simulink model "Ninebussys_Final"  (R2023b)
settings: Solver=FixedStepDiscrete  StartTime=0.0  StopTime=0.7  RelTol=1e-3
undefined symbols (not defined in the file or in its folder): D1, Delta
libraries: spsFourierLib x18, spsThreePhaseVIMeasurementLib x9, spsLoadFlowBusLib x9, spsPower3phInstantaneousLib x9, spsThreePhasePISectionLineLib x6, spsThreePhaseSeriesRLCLoadLib x4, spsThreePhaseTransformerTwoWindingsLib x3, spsSynchronousMachinepuStandardLib x3, spsThreePhaseParallelRLCLoadLib x3, spsExcitationSystemLib x3, spsGenericPowerSystemStabilizerLib x3, spsHydraulicTurbineandGovernorLib x3
settings Model: Creator=z0034ktr  LastModifiedBy=HP
settings SolverCC: AlgebraicLoopSolver=TrustRegion
settings DebuggingCC: UnconnectedInputMsg=warning  UnconnectedOutputMsg=warning  UnconnectedLineMsg=warning  ArithmeticOperatorsInVariantConditions=warning
settings ModelReferenceCC: EnableRefExpFcnMdlSchedulingChecks=on
settings SFSimCC: CustomCodeUndefinedFunction=UseInterfaceOnly

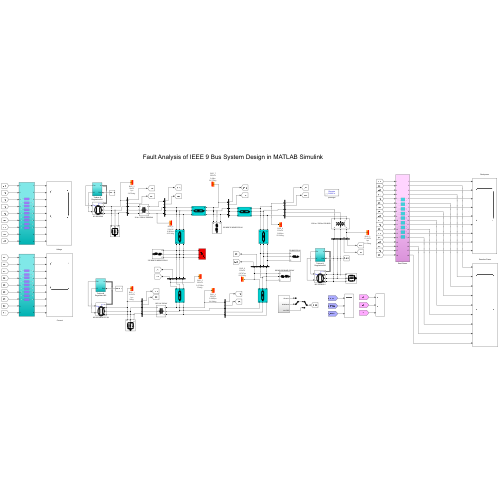
[thumbnail: Simulink's stored preview of the top-level diagram]
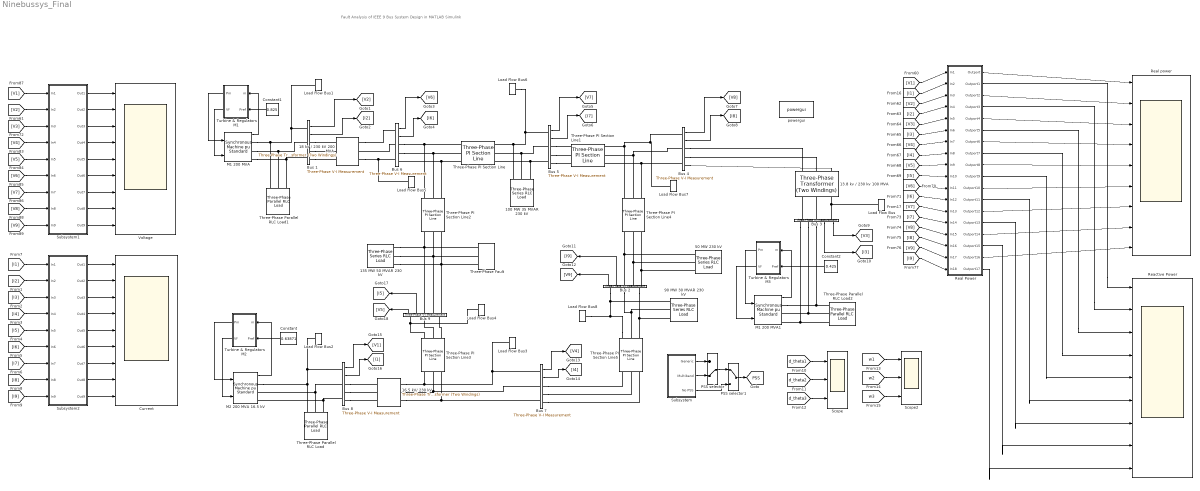
== system Ninebussys_Final ==
  note: Fault Analysis of IEEE 9 Bus System Design in MATLAB Simulink
  " Current" : Scope  NumInputPorts=9
  " Voltage" : Scope  NumInputPorts=9
  100 MW 35 MVAR 230 kV : spsThreePhaseSeriesRLCLoadLib/Three-Phase Series RLC Load  LConnTagsString=A|B|C  Configuration=Y (grounded)  NominalVoltage=(230000)*0.980041  Vabc=[1e3 1e3 1e3]  Vabcp=[1e3 1e3 1e3]  NominalFrequency=60  UnbalancedPower=off  ActivePower=100e6  InductivePower=35e6  CapacitivePower=0  Pabc=[10e3 9e3 11e3]  QLabc=[100 90 110]  QCabc=[100 90 110]  Pabcp=[10e3 9e3 11e3]  QLabcp=[100 90 110]  QCabcp=[100 90 110]  Measurements=None  LoadType=constant PQ
  13.8 kv / 230 kv 100 MVA : spsThreePhaseTransformerTwoWindingsLib/Three-Phase Transformer (Two Windings)  Winding1Connection=Delta (D1)  Winding2Connection=Yg  CoreType=Three single-phase transformers  SetSaturation=off  Hysteresis=off  DataFile='hysteresis'  SetInitialFlux=off  Measurements=None  UNITS=pu  NominalPower=[ 100e6 , 60 ]  Winding1=[ 13.8e3 , 0.002 , 0.08 ]  Winding2=[ 230e3 , 0.002 , 0.08 ]  Rm=500  Lm=500  L0=0.5  Saturation=[ 0,0 ; 0.0024,1.2 ; 1.0,1.52 ]  InitialFluxes=[ 0.8 , -0.8 , 0.7 ]  BreakLoop=off  DiscreteSolver=Trapezoidal iterative  DataType=off  TransfoNumber=1
  135 MW 50 MVAR 230 kV : spsThreePhaseSeriesRLCLoadLib/Three-Phase Series RLC Load  LConnTagsString=A|B|C  Configuration=Y (grounded)  NominalVoltage=(230000)*0.972469  Vabc=[1e3 1e3 1e3]  Vabcp=[1e3 1e3 1e3]  NominalFrequency=60  UnbalancedPower=off  ActivePower=135e6  InductivePower=50e6  CapacitivePower=0  Pabc=[10e3 9e3 11e3]  QLabc=[100 90 110]  QCabc=[100 90 110]  Pabcp=[10e3 9e3 11e3]  QLabcp=[100 90 110]  QCabcp=[100 90 110]  Measurements=None  LoadType=constant PQ
  16.5 kV/ 230 kV : spsThreePhaseTransformerTwoWindingsLib/Three-Phase Transformer (Two Windings)  Winding1Connection=Delta (D1)  Winding2Connection=Yg  CoreType=Three single-phase transformers  SetSaturation=off  Hysteresis=off  DataFile='hysteresis'  SetInitialFlux=off  Measurements=None  UNITS=pu  NominalPower=[ 200e6 , 60 ]  Winding1=[ 16.5e3 , 0.002 , 0.08 ]  Winding2=[ 230e3 , 0.002 , 0.08 ]  Rm=500  Lm=500  L0=0.5  Saturation=[ 0,0 ; 0.0024,1.2 ; 1.0,1.52 ]  InitialFluxes=[ 0.8 , -0.8 , 0.7 ]  BreakLoop=off  DiscreteSolver=Trapezoidal iterative  DataType=off  TransfoNumber=1
  18 kv / 230 kV 200 MVA : spsThreePhaseTransformerTwoWindingsLib/Three-Phase Transformer (Two Windings)  Winding1Connection=Delta (D1)  Winding2Connection=Yg  CoreType=Three single-phase transformers  SetSaturation=off  Hysteresis=off  DataFile='hysteresis'  SetInitialFlux=off  Measurements=None  UNITS=pu  NominalPower=[ 200e6 , 60 ]  Winding1=[ 18e3 , 0.002 , 0.08 ]  Winding2=[ 230e3 , 0.002 , 0.08 ]  Rm=500  Lm=500  L0=0.5  Saturation=[ 0,0 ; 0.0024,1.2 ; 1.0,1.52 ]  InitialFluxes=[ 0.8 , -0.8 , 0.7 ]  BreakLoop=off  DiscreteSolver=Trapezoidal iterative  DataType=off  TransfoNumber=1
  50 MW 230 kV : spsThreePhaseSeriesRLCLoadLib/Three-Phase Series RLC Load  LConnTagsString=A|B|C  Configuration=Y (grounded)  NominalVoltage=(230000)*0.978663  Vabc=[1e3 1e3 1e3]  Vabcp=[1e3 1e3 1e3]  NominalFrequency=60  UnbalancedPower=off  ActivePower=50e6  InductivePower=0  CapacitivePower=0  Pabc=[10e3 9e3 11e3]  QLabc=[100 90 110]  QCabc=[100 90 110]  Pabcp=[10e3 9e3 11e3]  QLabcp=[100 90 110]  QCabcp=[100 90 110]  Measurements=None  LoadType=constant PQ
  90 MW 30 MVAR 230 kV : spsThreePhaseSeriesRLCLoadLib/Three-Phase Series RLC Load  LConnTagsString=A|B|C  Configuration=Y (grounded)  NominalVoltage=(230000)*0.978663  Vabc=[1e3 1e3 1e3]  Vabcp=[1e3 1e3 1e3]  NominalFrequency=60  UnbalancedPower=off  ActivePower=90e6  InductivePower=30e6  CapacitivePower=0  Pabc=[10e3 9e3 11e3]  QLabc=[100 90 110]  QCabc=[100 90 110]  Pabcp=[10e3 9e3 11e3]  QLabcp=[100 90 110]  QCabcp=[100 90 110]  Measurements=None  LoadType=constant PQ
  Bus {1..9} (9 alike) : spsThreePhaseVIMeasurementLib/Three-Phase V-I Measurement  VoltageMeasurement=phase-to-ground  SetLabelV=off  LabelV=Vabc  Vpu=on  VpuLL=off  CurrentMeasurement=yes  SetLabelI=off  LabelI=Iabc  Ipu=on  Pbase=100e6  Vbase=500e3  OutputType=Complex  PhasorSimulation=off  PSBequivalent=0
  Constant : Constant  Value=0.63871
  Constant1 : Constant  Value=0.825
  Constant2 : Constant  Value=0.425
  Load Flow Bus : spsLoadFlowBusLib/Load Flow Bus  LConnTagsString=a  Phases=single  Connectors=on one side  ID=BUS_3  Vbase=13.8e3  Vref=1  Vangle=0  VLF=1  VLFb=1  VLFc=1  angleLF=3.115  angleLFb=0  angleLFc=0
  Load Flow Bus1 : spsLoadFlowBusLib/Load Flow Bus  LConnTagsString=a  Phases=single  Connectors=on one side  ID=BUS_2  Vbase=18e3  Vref=1  Vangle=0  VLF=1  VLFb=1  VLFc=1  angleLF=3.878  angleLFb=0  angleLFc=0
  Load Flow Bus2 : spsLoadFlowBusLib/Load Flow Bus  LConnTagsString=a  Phases=single  Connectors=on one side  ID=BUS_1  Vbase=16.5e3  Vref=1  Vangle=0  VLF=1  VLFb=1  VLFc=1  angleLF=0  angleLFb=0  angleLFc=0
  Load Flow Bus3 : spsLoadFlowBusLib/Load Flow Bus  LConnTagsString=a  Phases=single  Connectors=on one side  ID=BUS_4  Vbase=230e3  Vref=1  Vangle=0  VLF=0.9805  VLFb=1  VLFc=1  angleLF=24.06  angleLFb=0  angleLFc=0
  Load Flow Bus4 : spsLoadFlowBusLib/Load Flow Bus  LConnTagsString=a  Phases=single  Connectors=on one side  ID=BUS_5  Vbase=230e3  Vref=1  Vangle=0  VLF=0.9725  VLFb=1  VLFc=1  angleLF=23  angleLFb=0  angleLFc=0
  Load Flow Bus5 : spsLoadFlowBusLib/Load Flow Bus  LConnTagsString=a  Phases=single  Connectors=on one side  ID=BUS_6  Vbase=230e3  Vref=1  Vangle=0  VLF=0.9834  VLFb=1  VLFc=1  angleLF=26.21  angleLFb=0  angleLFc=0
  Load Flow Bus6 : spsLoadFlowBusLib/Load Flow Bus  LConnTagsString=a  Phases=single  Connectors=on one side  ID=BUS_7  Vbase=230e3  Vref=1  Vangle=0  VLF=0.98  VLFb=1  VLFc=1  angleLF=24.57  angleLFb=0  angleLFc=0
  Load Flow Bus7 : spsLoadFlowBusLib/Load Flow Bus  LConnTagsString=a  Phases=single  Connectors=on one side  ID=BUS_8  Vbase=230e3  Vref=1  Vangle=0  VLF=0.988  VLFb=1  VLFc=1  angleLF=25.24  angleLFb=0  angleLFc=0
  Load Flow Bus8 : spsLoadFlowBusLib/Load Flow Bus  LConnTagsString=a  Phases=single  Connectors=on one side  ID=BUS_9  Vbase=230e3  Vref=1  Vangle=0  VLF=0.9787  VLFb=1  VLFc=1  angleLF=22.61  angleLFb=0  angleLFc=0
  M1 200 MVA : spsSynchronousMachinepuStandardLib/Synchronous Machine pu Standard  PresetModel=No  MechanicalLoad=Mechanical power Pm  ShowDetailedParameters=on  RotorType=Salient-pole  Units=per unit standard parameters  MeasurementBus=off  NominalParameters="[200E6  18000   60 ]"  Reactances1=[ 31 32 33 34 35 36 37 ]  Reactances2=[ 1.305, 0.296, 0.252, 0.474, 0.243, 0.18 ]  dAxisTimeConstants=Short-circuit  qAxisTimeConstants=Open-circuit  TimeConstants1=[]  TimeConstants2=[]  TimeConstants3=[]  TimeConstants4=[]  TimeConstants5=[ 1.01, 0.053, 0.1 ]  TimeConstants6=[]  TimeConstants7=[]  TimeConstants8=[]  StatorResistance=2.8544e-3  Mechanical="[ 3.7 0  32]"  PolePairs=32  InitialConditions=[0 -66.0372 0.836682 0.836682 0.836682 -5.70736 -125.707 114.293 1.48174]  SetSaturation=off  Saturation=[0.6404,0.7127,0.8441,0.9214,0.9956,1.082,1.19,1.316,1.457;0.7,0.7698,0.8872,0.9466,0.9969,1.046,1.1,1.151,1.201]  LoadFlowParameters=[1 950000000 0 0]  TsPowergui=0  TsBlock=-1  IterativeModel=Trapezoidal non iterative  IterativeDiscreteModel=Trapezoidal non iterative  BusType=PV  Pref=165e6  Qref=0  Qmin=-Inf  Qmax=Inf  PLF=0  QLF=0
  M1 200 MVA1 : spsSynchronousMachinepuStandardLib/Synchronous Machine pu Standard  PresetModel=No  MechanicalLoad=Mechanical power Pm  ShowDetailedParameters=on  RotorType=Salient-pole  Units=per unit standard parameters  MeasurementBus=off  NominalParameters="[200E6  18000   60 ]"  Reactances1=[ 31 32 33 34 35 36 37 ]  Reactances2=[ 1.305, 0.296, 0.252, 0.474, 0.243, 0.18 ]  dAxisTimeConstants=Short-circuit  qAxisTimeConstants=Open-circuit  TimeConstants1=[]  TimeConstants2=[]  TimeConstants3=[]  TimeConstants4=[]  TimeConstants5=[ 1.01, 0.053, 0.1 ]  TimeConstants6=[]  TimeConstants7=[]  TimeConstants8=[]  StatorResistance=2.8544e-3  Mechanical="[ 3.7 0  32]"  PolePairs=32  InitialConditions=[0 -68.7855 0.55925 0.55925 0.55925 -4.47761 -124.478 115.522 1.04657]  SetSaturation=off  Saturation=[0.6404,0.7127,0.8441,0.9214,0.9956,1.082,1.19,1.316,1.457;0.7,0.7698,0.8872,0.9466,0.9969,1.046,1.1,1.151,1.201]  LoadFlowParameters=[1 950000000 0 0]  TsPowergui=0  TsBlock=-1  IterativeModel=Trapezoidal non iterative  IterativeDiscreteModel=Trapezoidal non iterative  BusType=PV  Pref=85e6  Qref=0  Qmin=-Inf  Qmax=Inf  PLF=0  QLF=0
  M2 200 MVA 16.5 kV : spsSynchronousMachinepuStandardLib/Synchronous Machine pu Standard  PresetModel=No  MechanicalLoad=Mechanical power Pm  ShowDetailedParameters=on  RotorType=Salient-pole  Units=per unit standard parameters  MeasurementBus=off  NominalParameters="[200E6  16500   60 ]"  Reactances1=[ 31 32 33 34 35 36 37 ]  Reactances2=[ 1.305, 0.296, 0.252, 0.474, 0.243, 0.18 ]  dAxisTimeConstants=Short-circuit  qAxisTimeConstants=Open-circuit  TimeConstants1=[]  TimeConstants2=[]  TimeConstants3=[]  TimeConstants4=[]  TimeConstants5=[ 1.01, 0.053, 0.1 ]  TimeConstants6=[]  TimeConstants7=[]  TimeConstants8=[]  StatorResistance=2.8544e-3  Mechanical="[ 3.7 0  32]"  PolePairs=32  InitialConditions=[0 -74.1936 0.653801 0.653801 0.653801 -12.3345 -132.335 107.665 1.36624]  SetSaturation=off  Saturation=[0.6404,0.7127,0.8441,0.9214,0.9956,1.082,1.19,1.316,1.457;0.7,0.7698,0.8872,0.9466,0.9969,1.046,1.1,1.151,1.201]  LoadFlowParameters=[2 4000000000 0 0]  TsPowergui=0  TsBlock=-1  IterativeModel=Trapezoidal non iterative  IterativeDiscreteModel=Trapezoidal non iterative  BusType=swing  Pref=0  Qref=0  Qmin=-Inf  Qmax=Inf  PLF=0  QLF=0
  PSS selector : ManualSwitch  CurrentSetting=0
  PSS selector1 : ManualSwitch
  "Reactive Power " : Scope  NumInputPorts=9
  Real Power : Subsystem
  "Real power " : Scope  NumInputPorts=9
  Scope : Scope  NumInputPorts=3
  Scope2 : Scope  NumInputPorts=3
  Subsystem : Subsystem
  Subsystem1 : Subsystem
  Subsystem2 : Subsystem
  Three-Phase PI Section Line : spsThreePhasePISectionLineLib/Three-Phase PI Section Line  LConnTagsString=a|b|c  RConnTagsString=A|B|C  Length=50  Frequency=60  Resistances=[ 0.01273 0.3864]  Inductances="[ 0.9337e-3  4.1264e-3]"  Capacitances=[12.74e-9 7.751e-9]
  Three-Phase PI Section Line1 : spsThreePhasePISectionLineLib/Three-Phase PI Section Line  LConnTagsString=a|b|c  RConnTagsString=A|B|C  Length=100  Frequency=60  Resistances=[ 0.01273 0.3864]  Inductances="[ 0.9337e-3  4.1264e-3]"  Capacitances=[12.74e-9 7.751e-9]
  Three-Phase PI Section Line2 : spsThreePhasePISectionLineLib/Three-Phase PI Section Line  LConnTagsString=a|b|c  RConnTagsString=A|B|C  Length=100  Frequency=60  Resistances=[ 0.01273 0.3864]  Inductances="[ 0.9337e-3  4.1264e-3]"  Capacitances=[12.74e-9 7.751e-9]
  Three-Phase PI Section Line3 : spsThreePhasePISectionLineLib/Three-Phase PI Section Line  LConnTagsString=a|b|c  RConnTagsString=A|B|C  Length=50  Frequency=60  Resistances=[ 0.01273 0.3864]  Inductances="[ 0.9337e-3  4.1264e-3]"  Capacitances=[12.74e-9 7.751e-9]
  Three-Phase PI Section Line4 : spsThreePhasePISectionLineLib/Three-Phase PI Section Line  LConnTagsString=a|b|c  RConnTagsString=A|B|C  Length=100  Frequency=60  Resistances=[ 0.01273 0.3864]  Inductances="[ 0.9337e-3  4.1264e-3]"  Capacitances=[12.74e-9 7.751e-9]
  Three-Phase PI Section Line5 : spsThreePhasePISectionLineLib/Three-Phase PI Section Line  LConnTagsString=a|b|c  RConnTagsString=A|B|C  Length=50  Frequency=60  Resistances=[ 0.01273 0.3864]  Inductances="[ 0.9337e-3  4.1264e-3]"  Capacitances=[12.74e-9 7.751e-9]
  Three-Phase Parallel RLC Load : spsThreePhaseParallelRLCLoadLib/Three-Phase Parallel RLC Load  LConnTagsString=A|B|C  Configuration=Y (grounded)  NominalVoltage=16.5e3  Vabc=[1e3 1e3 1e3]  Vabcp=[1e3 1e3 1e3]  NominalFrequency=60  UnbalancedPower=off  ActivePower=10e3  InductivePower=100  CapacitivePower=100  Pabc=[10e3 9e3 11e3]  QLabc=[100 90 110]  QCabc=[100 90 110]  Pabcp=[10e3 9e3 11e3]  QLabcp=[100 90 110]  QCabcp=[100 90 110]  Measurements=None  LoadType=constant Z
  Three-Phase Parallel RLC Load1 : spsThreePhaseParallelRLCLoadLib/Three-Phase Parallel RLC Load  LConnTagsString=A|B|C  Configuration=Y (grounded)  NominalVoltage=18e3  Vabc=[1e3 1e3 1e3]  Vabcp=[1e3 1e3 1e3]  NominalFrequency=60  UnbalancedPower=off  ActivePower=10e3  InductivePower=100  CapacitivePower=100  Pabc=[10e3 9e3 11e3]  QLabc=[100 90 110]  QCabc=[100 90 110]  Pabcp=[10e3 9e3 11e3]  QLabcp=[100 90 110]  QCabcp=[100 90 110]  Measurements=None  LoadType=constant Z
  Three-Phase Parallel RLC Load2 : spsThreePhaseParallelRLCLoadLib/Three-Phase Parallel RLC Load  LConnTagsString=A|B|C  Configuration=Y (grounded)  NominalVoltage=13.8e3  Vabc=[1e3 1e3 1e3]  Vabcp=[1e3 1e3 1e3]  NominalFrequency=60  UnbalancedPower=off  ActivePower=10e3  InductivePower=100  CapacitivePower=100  Pabc=[10e3 9e3 11e3]  QLabc=[100 90 110]  QCabc=[100 90 110]  Pabcp=[10e3 9e3 11e3]  QLabcp=[100 90 110]  QCabcp=[100 90 110]  Measurements=None  LoadType=constant Z
  Three-Phase Fault : spsThreePhaseFaultLib/Three-Phase Fault  InitialStates=0  FaultA=on  FaultB=on  FaultC=on  GroundFault=on  SwitchTimes=[0.4 0.5]  External=off  SwitchStatus=NaN  FaultResistance=0.001  GroundResistance=0.01  SnubberResistance=1e6  SnubberCapacitance=inf  Measurements=None
  Turbine & Regulators M1 : Subsystem
  Turbine & Regulators M2 : Subsystem
  Turbine & Regulators M3 : Subsystem
  powergui : sps_lib/powergui  Priority=1  SimulationMode=Discrete  SampleTime=50e-5  frequency=60  Iterations=50  frequencyindice=0  Pbase=200  ErrMax=0.0001  UnitsV=kV  UnitsW=MW  buscounter=0  FunctionMessages=off  echomessages=off  EnableUseOfTLC=off  CurrentSourceSwitches=off  DisableSnubberDevices=off  DisableRonSwitches=off  DisableVfSwitches=off  DisplayEquations=off  AutomaticDiscreteSolvers=off  SolverType=Backward Euler  Interpol=off  ExternalGateDelay=off  methode=off  Ts=100  x0status=blocks  SPID=on  SwTol=0  HookPort=off  NonlinearTolerance=1e-4  nMaxIteration=100  ContinueOnMaxIteration=off  RestoreLinks=warning  ResistiveCurrentMeasurement=off  Frange=[0:2:500]  Ylog=off  Xlog=on  ShowGrid=off  save=off  variable=ZData  structure=0  ZoomFFT=off  StartTime=0.0  cycles=1  DisplayStyle=1  fundamental=60  FreqAxis=off  MaxFrequency=1000  frequencyindicesteady=1  RmsSteady=1  display=off
  tag scope: PSS=global
  wires:
  M2 200 MVA 16.5 kV/1 -> Turbine & Regulators M2/1(m)
  Turbine & Regulators M2/2(Vf) -> M2 200 MVA 16.5 kV/2
  Turbine & Regulators M2/1(Pm) -> M2 200 MVA 16.5 kV/1
  Constant/1 -> Turbine & Regulators M2/2(Pref)
  PSS selector/1 -> PSS selector1/1
  Subsystem/1(Generic) -> PSS selector/1
  Subsystem/3(No PSS) -> PSS selector1/2
  Subsystem/2(Multiband) -> PSS selector/2
  PSS selector1/1 -> [PSS]
  M1 200 MVA/1 -> Turbine & Regulators M1/1(m)
  Constant1/1 -> Turbine & Regulators M1/2(Pref)
  Turbine & Regulators M1/1(Pm) -> M1 200 MVA/1
  Turbine & Regulators M1/2(Vf) -> M1 200 MVA/2
  Turbine & Regulators M3/2(Vf) -> M1 200 MVA1/2
  Turbine & Regulators M3/1(Pm) -> M1 200 MVA1/1
  M1 200 MVA1/1 -> Turbine & Regulators M3/1(m)
  Constant2/1 -> Turbine & Regulators M3/2(Pref)
  Bus 1/1 -> [V2]
  Bus 1/2 -> [I2]
  Bus 6/1 -> [V6]
  Bus 6/2 -> [I6]
  Bus 5/1 -> [V7]
  Bus 5/2 -> [I7]
  Bus 4/1 -> [V8]
  Bus 4/2 -> [I8]
  Bus 3/1 -> [V3]
  Bus 3/2 -> [I3]
  Bus 2/1 -> [V9]
  Bus 2/2 -> [I9]
  Bus 7/1 -> [V4]
  Bus 7/2 -> [I4]
  Bus 8/2 -> [I1]
  Bus 8/1 -> [V1]
  Bus 9/1 -> [V5]
  Bus 9/2 -> [I5]
  Subsystem1/4(Out4) -> " Voltage"/4
  Subsystem1/2(Out2) -> " Voltage"/2
  [V6] -> Subsystem1/6(In6)
  [V3] -> Subsystem1/3(In3)
  [V1] -> Subsystem1/1(In1)
  Subsystem1/7(Out7) -> " Voltage"/7
  [V9] -> Subsystem1/9(In9)
  [V5] -> Subsystem1/5(In5)
  Subsystem1/9(Out9) -> " Voltage"/9
  [V8] -> Subsystem1/8(In8)
  Subsystem1/6(Out6) -> " Voltage"/6
  [V7] -> Subsystem1/7(In7)
  Subsystem1/8(Out8) -> " Voltage"/8
  Subsystem1/5(Out5) -> " Voltage"/5
  Subsystem1/1(Out1) -> " Voltage"/1
  [V2] -> Subsystem1/2(In2)
  [V4] -> Subsystem1/4(In4)
  Subsystem1/3(Out3) -> " Voltage"/3
  Subsystem2/3(Out3) -> " Current"/3
  [I4] -> Subsystem2/4(In4)
  [I2] -> Subsystem2/2(In2)
  Subsystem2/1(Out1) -> " Current"/1
  [I7] -> Subsystem2/7(In7)
  Subsystem2/5(Out5) -> " Current"/5
  Subsystem2/8(Out8) -> " Current"/8
  Subsystem2/6(Out6) -> " Current"/6
  [I8] -> Subsystem2/8(In8)
  [I5] -> Subsystem2/5(In5)
  Subsystem2/7(Out7) -> " Current"/7
  [I3] -> Subsystem2/3(In3)
  [I6] -> Subsystem2/6(In6)
  [I9] -> Subsystem2/9(In9)
  [I1] -> Subsystem2/1(In1)
  Subsystem2/9(Out9) -> " Current"/9
  Subsystem2/2(Out2) -> " Current"/2
  Subsystem2/4(Out4) -> " Current"/4
  [d_theta1] -> Scope/1
  [w1] -> Scope2/1
  [w2] -> Scope2/2
  [w3] -> Scope2/3
  [V3] -> Real Power/5(In5)
  [I2] -> Real Power/4(In4)
  [I9] -> Real Power/18(In18)
  Real Power/8(Outport7) -> "Reactive Power "/4
  Real Power/7(Outport6) -> "Real power "/4
  [V4] -> Real Power/7(In7)
  Real Power/5(Outport4) -> "Real power "/3
  Real Power/6(Outport5) -> "Reactive Power "/3
  [I3] -> Real Power/6(In6)
  [I5] -> Real Power/10(In10)
  [I4] -> Real Power/8(In8)
  [I8] -> Real Power/16(In16)
  [I1] -> Real Power/2(In2)
  Real Power/2(Outport1) -> "Reactive Power "/1
  [V6] -> Real Power/11(In11)
  [V1] -> Real Power/1(In1)
  Real Power/1(Outport) -> "Real power "/1
  Real Power/4(Outport3) -> "Reactive Power "/2
  [V9] -> Real Power/17(In17)
  Real Power/16(Outport15) -> "Reactive Power "/8
  [V5] -> Real Power/9(In9)
  [V7] -> Real Power/13(In13)
  Real Power/18(Outport17) -> "Reactive Power "/9
  Real Power/17(Outport16) -> "Real power "/9
  [V8] -> Real Power/15(In15)
  Real Power/3(Outport2) -> "Real power "/2
  Real Power/14(Outport13) -> "Reactive Power "/7
  Real Power/9(Outport8) -> "Real power "/5
  Real Power/15(Outport14) -> "Real power "/8
  Real Power/13(Outport12) -> "Real power "/7
  [I7] -> Real Power/14(In14)
  Real Power/12(Outport11) -> "Reactive Power "/6
  Real Power/10(Outport9) -> "Reactive Power "/5
  [V2] -> Real Power/3(In3)
  Real Power/11(Outport10) -> "Real power "/6
  [I6] -> Real Power/12(In12)
  [d_theta2] -> Scope/2
  [d_theta3] -> Scope/3
  connections:
  16.5 kV/ 230 kV/RConn1 -- Bus 7/LConn1 -- Load Flow Bus3/LConn1 -- Three-Phase PI Section Line3/RConn1
  16.5 kV/ 230 kV/RConn2 -- Bus 7/LConn2 -- Three-Phase PI Section Line3/RConn2
  16.5 kV/ 230 kV/RConn3 -- Bus 7/LConn3 -- Three-Phase PI Section Line3/RConn3
  50 MW 230 kV/LConn1 -- Bus 2/RConn1 -- Three-Phase PI Section Line4/RConn1
  Bus 2/LConn3 -- Three-Phase PI Section Line5/LConn3 -- 90 MW 30 MVAR 230 kV/LConn3
  Three-Phase PI Section Line4/LConn1 -- Bus 4/LConn1 -- Load Flow Bus7/LConn1 -- Three-Phase PI Section Line1/RConn1
  Three-Phase PI Section Line4/LConn2 -- Bus 4/LConn2 -- Three-Phase PI Section Line1/RConn2
  Three-Phase PI Section Line4/LConn3 -- Bus 4/LConn3 -- Three-Phase PI Section Line1/RConn3
  Bus 5/RConn1 -- Three-Phase PI Section Line1/LConn1
  Bus 5/LConn2 -- 100 MW 35 MVAR 230 kV/LConn2 -- Three-Phase PI Section Line/RConn2
  Bus 5/LConn3 -- 100 MW 35 MVAR 230 kV/LConn3 -- Three-Phase PI Section Line/RConn3
  135 MW 50 MVAR 230 kV/LConn1 -- Bus 9/RConn1 -- Three-Phase Fault/LConn1 -- Three-Phase PI Section Line2/RConn1
  135 MW 50 MVAR 230 kV/LConn3 -- Bus 9/RConn3 -- Three-Phase Fault/LConn3 -- Three-Phase PI Section Line2/RConn3
  Three-Phase PI Section Line2/LConn3 -- Three-Phase PI Section Line/LConn3 -- Bus 6/RConn3
  Three-Phase PI Section Line2/LConn2 -- Three-Phase PI Section Line/LConn2 -- Bus 6/RConn2
  Bus 6/RConn1 -- Three-Phase PI Section Line/LConn1 -- Three-Phase PI Section Line2/LConn1
  Three-Phase Parallel RLC Load2/LConn2 -- M1 200 MVA1/RConn2 -- Bus 3/RConn2
  Three-Phase Parallel RLC Load2/LConn3 -- M1 200 MVA1/RConn3 -- Bus 3/RConn3
  Three-Phase Parallel RLC Load/LConn1 -- M2 200 MVA 16.5 kV/RConn1 -- Bus 8/LConn1 -- Load Flow Bus2/LConn1
  Three-Phase Parallel RLC Load/LConn2 -- Bus 8/LConn2 -- M2 200 MVA 16.5 kV/RConn2
  Three-Phase Parallel RLC Load/LConn3 -- Bus 8/LConn3 -- M2 200 MVA 16.5 kV/RConn3
  50 MW 230 kV/LConn3 -- Bus 2/RConn3 -- Three-Phase PI Section Line4/RConn3
  Bus 2/LConn2 -- Three-Phase PI Section Line5/LConn2 -- 90 MW 30 MVAR 230 kV/LConn2
  Three-Phase PI Section Line5/LConn1 -- Bus 2/LConn1 -- 90 MW 30 MVAR 230 kV/LConn1 -- Load Flow Bus8/LConn1
  50 MW 230 kV/LConn2 -- Bus 2/RConn2 -- Three-Phase PI Section Line4/RConn2
  Bus 1/RConn3 -- 18 kv / 230 kV 200 MVA/LConn3
  Bus 1/RConn2 -- 18 kv / 230 kV 200 MVA/LConn2
  Bus 1/RConn1 -- 18 kv / 230 kV 200 MVA/LConn1
  M1 200 MVA/RConn3 -- Bus 1/LConn3 -- Three-Phase Parallel RLC Load1/LConn3
  M1 200 MVA/RConn2 -- Bus 1/LConn2 -- Three-Phase Parallel RLC Load1/LConn2
  M1 200 MVA/RConn1 -- Bus 1/LConn1 -- Load Flow Bus1/LConn1 -- Three-Phase Parallel RLC Load1/LConn1
  Bus 6/LConn2 -- 18 kv / 230 kV 200 MVA/RConn2
  18 kv / 230 kV 200 MVA/RConn3 -- Load Flow Bus5/LConn1 -- Bus 6/LConn3
  18 kv / 230 kV 200 MVA/RConn1 -- Bus 6/LConn1
  100 MW 35 MVAR 230 kV/LConn1 -- Load Flow Bus6/LConn1 -- Bus 5/LConn1 -- Three-Phase PI Section Line/RConn1
  Bus 5/RConn2 -- Three-Phase PI Section Line1/LConn2
  Bus 5/RConn3 -- Three-Phase PI Section Line1/LConn3
  Bus 4/RConn3 -- 13.8 kv / 230 kv 100 MVA/RConn3
  Bus 4/RConn2 -- 13.8 kv / 230 kv 100 MVA/RConn2
  Bus 4/RConn1 -- 13.8 kv / 230 kv 100 MVA/RConn1
  Bus 3/LConn3 -- 13.8 kv / 230 kv 100 MVA/LConn1
  Bus 3/LConn2 -- 13.8 kv / 230 kv 100 MVA/LConn2
  Bus 3/LConn1 -- Load Flow Bus/LConn1 -- 13.8 kv / 230 kv 100 MVA/LConn3
  M1 200 MVA1/RConn1 -- Bus 3/RConn1 -- Three-Phase Parallel RLC Load2/LConn1
  Bus 7/RConn1 -- Three-Phase PI Section Line5/RConn1
  Bus 7/RConn2 -- Three-Phase PI Section Line5/RConn2
  Bus 7/RConn3 -- Three-Phase PI Section Line5/RConn3
  Bus 8/RConn3 -- 16.5 kV/ 230 kV/LConn3
  Bus 8/RConn2 -- 16.5 kV/ 230 kV/LConn2
  Bus 8/RConn1 -- 16.5 kV/ 230 kV/LConn1
  135 MW 50 MVAR 230 kV/LConn2 -- Bus 9/RConn2 -- Three-Phase Fault/LConn2 -- Three-Phase PI Section Line2/RConn2
  Three-Phase PI Section Line3/LConn3 -- Bus 9/LConn3
  Three-Phase PI Section Line3/LConn2 -- Bus 9/LConn2
  Three-Phase PI Section Line3/LConn1 -- Load Flow Bus4/LConn1 -- Bus 9/LConn1

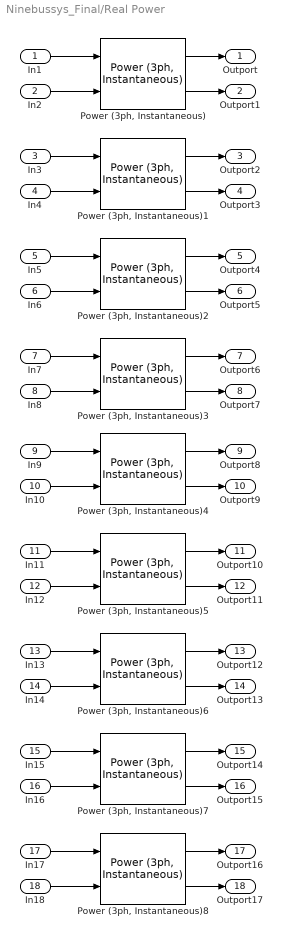
== system Ninebussys_Final/Real Power ==
  In1 : Inport
  In2 : Inport  Port=2
  In3 : Inport  Port=3
  In4 : Inport  Port=4
  In5 : Inport  Port=5
  In6 : Inport  Port=6
  In7 : Inport  Port=7
  In8 : Inport  Port=8
  In9 : Inport  Port=9
  In10 : Inport  Port=10
  In11 : Inport  Port=11
  In12 : Inport  Port=12
  In13 : Inport  Port=13
  In14 : Inport  Port=14
  In15 : Inport  Port=15
  In16 : Inport  Port=16
  In17 : Inport  Port=17
  In18 : Inport  Port=18
  Power (3ph, Instantaneous){,1..8} (9 alike) : spsPower3phInstantaneousLib/Power (3ph, Instantaneous)
  Outport : Outport  VectorParamsAs1DForOutWhenUnconnected=off
  Outport1 : Outport  Port=2  VectorParamsAs1DForOutWhenUnconnected=off
  Outport2 : Outport  Port=3  VectorParamsAs1DForOutWhenUnconnected=off
  Outport3 : Outport  Port=4  VectorParamsAs1DForOutWhenUnconnected=off
  Outport4 : Outport  Port=5  VectorParamsAs1DForOutWhenUnconnected=off
  Outport5 : Outport  Port=6  VectorParamsAs1DForOutWhenUnconnected=off
  Outport6 : Outport  Port=7  VectorParamsAs1DForOutWhenUnconnected=off
  Outport7 : Outport  Port=8  VectorParamsAs1DForOutWhenUnconnected=off
  Outport8 : Outport  Port=9  VectorParamsAs1DForOutWhenUnconnected=off
  Outport9 : Outport  Port=10  VectorParamsAs1DForOutWhenUnconnected=off
  Outport10 : Outport  Port=11  VectorParamsAs1DForOutWhenUnconnected=off
  Outport11 : Outport  Port=12  VectorParamsAs1DForOutWhenUnconnected=off
  Outport12 : Outport  Port=13  VectorParamsAs1DForOutWhenUnconnected=off
  Outport13 : Outport  Port=14  VectorParamsAs1DForOutWhenUnconnected=off
  Outport14 : Outport  Port=15  VectorParamsAs1DForOutWhenUnconnected=off
  Outport15 : Outport  Port=16  VectorParamsAs1DForOutWhenUnconnected=off
  Outport16 : Outport  Port=17  VectorParamsAs1DForOutWhenUnconnected=off
  Outport17 : Outport  Port=18  VectorParamsAs1DForOutWhenUnconnected=off
  wires:
  In1/1 -> "Power (3ph, Instantaneous)"/1
  In2/1 -> "Power (3ph, Instantaneous)"/2
  "Power (3ph, Instantaneous)"/1 -> Outport/1
  "Power (3ph, Instantaneous)"/2 -> Outport1/1
  "Power (3ph, Instantaneous)1"/2 -> Outport3/1
  "Power (3ph, Instantaneous)1"/1 -> Outport2/1
  In4/1 -> "Power (3ph, Instantaneous)1"/2
  In3/1 -> "Power (3ph, Instantaneous)1"/1
  In7/1 -> "Power (3ph, Instantaneous)3"/1
  In8/1 -> "Power (3ph, Instantaneous)3"/2
  "Power (3ph, Instantaneous)3"/1 -> Outport6/1
  "Power (3ph, Instantaneous)3"/2 -> Outport7/1
  "Power (3ph, Instantaneous)2"/2 -> Outport5/1
  "Power (3ph, Instantaneous)2"/1 -> Outport4/1
  In6/1 -> "Power (3ph, Instantaneous)2"/2
  In5/1 -> "Power (3ph, Instantaneous)2"/1
  In13/1 -> "Power (3ph, Instantaneous)6"/1
  In14/1 -> "Power (3ph, Instantaneous)6"/2
  "Power (3ph, Instantaneous)6"/1 -> Outport12/1
  "Power (3ph, Instantaneous)6"/2 -> Outport13/1
  "Power (3ph, Instantaneous)7"/2 -> Outport15/1
  "Power (3ph, Instantaneous)7"/1 -> Outport14/1
  In16/1 -> "Power (3ph, Instantaneous)7"/2
  In15/1 -> "Power (3ph, Instantaneous)7"/1
  In11/1 -> "Power (3ph, Instantaneous)5"/1
  In12/1 -> "Power (3ph, Instantaneous)5"/2
  "Power (3ph, Instantaneous)5"/1 -> Outport10/1
  "Power (3ph, Instantaneous)5"/2 -> Outport11/1
  "Power (3ph, Instantaneous)4"/2 -> Outport9/1
  "Power (3ph, Instantaneous)4"/1 -> Outport8/1
  In10/1 -> "Power (3ph, Instantaneous)4"/2
  In9/1 -> "Power (3ph, Instantaneous)4"/1
  In17/1 -> "Power (3ph, Instantaneous)8"/1
  In18/1 -> "Power (3ph, Instantaneous)8"/2
  "Power (3ph, Instantaneous)8"/1 -> Outport16/1
  "Power (3ph, Instantaneous)8"/2 -> Outport17/1

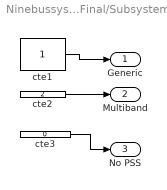
== system Ninebussys_Final/Subsystem ==
  cte1 : Constant
  cte2 : Constant  Value=2
  cte3 : Constant  Value=0
  Generic : Outport  VectorParamsAs1DForOutWhenUnconnected=off
  Multiband : Outport  Port=2  VectorParamsAs1DForOutWhenUnconnected=off
  No PSS : Outport  Port=3  VectorParamsAs1DForOutWhenUnconnected=off
  wires:
  cte1/1 -> Generic/1
  cte2/1 -> Multiband/1
  cte3/1 -> No PSS/1

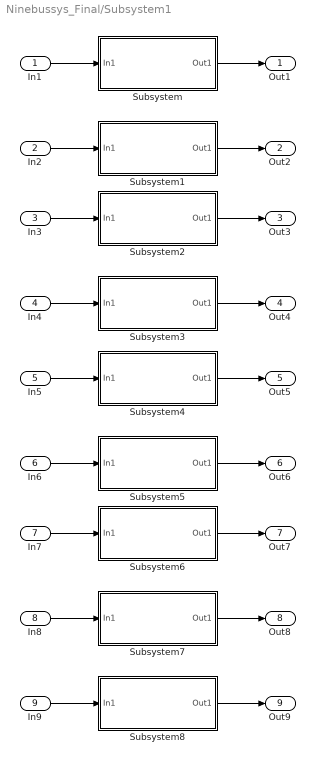
== system Ninebussys_Final/Subsystem1 ==
  In1 : Inport
  In2 : Inport  Port=2
  In3 : Inport  Port=3
  In4 : Inport  Port=4
  In5 : Inport  Port=5
  In6 : Inport  Port=6
  In7 : Inport  Port=7
  In8 : Inport  Port=8
  In9 : Inport  Port=9
  Subsystem : Subsystem
  Subsystem1 : Subsystem
  Subsystem2 : Subsystem
  Subsystem3 : Subsystem
  Subsystem4 : Subsystem
  Subsystem5 : Subsystem
  Subsystem6 : Subsystem
  Subsystem7 : Subsystem
  Subsystem8 : Subsystem
  Out1 : Outport  VectorParamsAs1DForOutWhenUnconnected=off
  Out2 : Outport  Port=2  VectorParamsAs1DForOutWhenUnconnected=off
  Out3 : Outport  Port=3  VectorParamsAs1DForOutWhenUnconnected=off
  Out4 : Outport  Port=4  VectorParamsAs1DForOutWhenUnconnected=off
  Out5 : Outport  Port=5  VectorParamsAs1DForOutWhenUnconnected=off
  Out6 : Outport  Port=6  VectorParamsAs1DForOutWhenUnconnected=off
  Out7 : Outport  Port=7  VectorParamsAs1DForOutWhenUnconnected=off
  Out8 : Outport  Port=8  VectorParamsAs1DForOutWhenUnconnected=off
  Out9 : Outport  Port=9  VectorParamsAs1DForOutWhenUnconnected=off
  wires:
  In1/1 -> Subsystem/1(In1)
  Subsystem/1(Out1) -> Out1/1
  Subsystem1/1(Out1) -> Out2/1
  In2/1 -> Subsystem1/1(In1)
  In4/1 -> Subsystem3/1(In1)
  Subsystem3/1(Out1) -> Out4/1
  Subsystem2/1(Out1) -> Out3/1
  In3/1 -> Subsystem2/1(In1)
  In7/1 -> Subsystem6/1(In1)
  Subsystem6/1(Out1) -> Out7/1
  Subsystem7/1(Out1) -> Out8/1
  In8/1 -> Subsystem7/1(In1)
  In6/1 -> Subsystem5/1(In1)
  Subsystem5/1(Out1) -> Out6/1
  Subsystem4/1(Out1) -> Out5/1
  In5/1 -> Subsystem4/1(In1)
  In9/1 -> Subsystem8/1(In1)
  Subsystem8/1(Out1) -> Out9/1

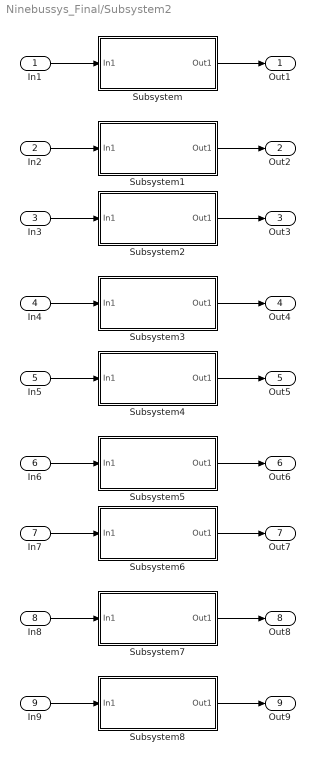
== system Ninebussys_Final/Subsystem2 ==
  In1 : Inport
  In2 : Inport  Port=2
  In3 : Inport  Port=3
  In4 : Inport  Port=4
  In5 : Inport  Port=5
  In6 : Inport  Port=6
  In7 : Inport  Port=7
  In8 : Inport  Port=8
  In9 : Inport  Port=9
  Subsystem : Subsystem
  Subsystem1 : Subsystem
  Subsystem2 : Subsystem
  Subsystem3 : Subsystem
  Subsystem4 : Subsystem
  Subsystem5 : Subsystem
  Subsystem6 : Subsystem
  Subsystem7 : Subsystem
  Subsystem8 : Subsystem
  Out1 : Outport  VectorParamsAs1DForOutWhenUnconnected=off
  Out2 : Outport  Port=2  VectorParamsAs1DForOutWhenUnconnected=off
  Out3 : Outport  Port=3  VectorParamsAs1DForOutWhenUnconnected=off
  Out4 : Outport  Port=4  VectorParamsAs1DForOutWhenUnconnected=off
  Out5 : Outport  Port=5  VectorParamsAs1DForOutWhenUnconnected=off
  Out6 : Outport  Port=6  VectorParamsAs1DForOutWhenUnconnected=off
  Out7 : Outport  Port=7  VectorParamsAs1DForOutWhenUnconnected=off
  Out8 : Outport  Port=8  VectorParamsAs1DForOutWhenUnconnected=off
  Out9 : Outport  Port=9  VectorParamsAs1DForOutWhenUnconnected=off
  wires:
  Subsystem8/1(Out1) -> Out9/1
  In9/1 -> Subsystem8/1(In1)
  In5/1 -> Subsystem4/1(In1)
  Subsystem4/1(Out1) -> Out5/1
  Subsystem5/1(Out1) -> Out6/1
  In6/1 -> Subsystem5/1(In1)
  In8/1 -> Subsystem7/1(In1)
  Subsystem7/1(Out1) -> Out8/1
  Subsystem6/1(Out1) -> Out7/1
  In7/1 -> Subsystem6/1(In1)
  In3/1 -> Subsystem2/1(In1)
  Subsystem2/1(Out1) -> Out3/1
  Subsystem3/1(Out1) -> Out4/1
  In4/1 -> Subsystem3/1(In1)
  In2/1 -> Subsystem1/1(In1)
  Subsystem1/1(Out1) -> Out2/1
  Subsystem/1(Out1) -> Out1/1
  In1/1 -> Subsystem/1(In1)

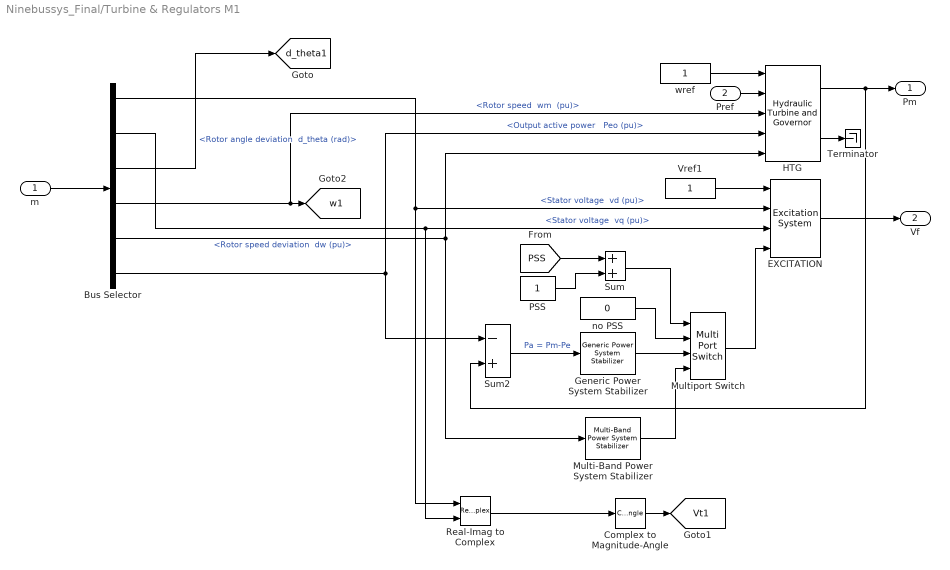
== system Ninebussys_Final/Turbine & Regulators M1 ==
  m : Inport
  Pref : Inport  Port=2
  Bus Selector : BusSelector  OutputSignals="dq0 components.Stator voltage  vd (pu),dq0 components.Stator voltage  vq (pu),Mechanical.Rotor angle deviation  d_theta (rad),Mechanical.Rotor speed  wm  (pu),Mechanical.Rotor speed deviation  dw (pu),Output active power   Peo (pu)"
  Complex to Magnitude-Angle : ComplexToMagnitudeAngle  Output=Magnitude
  EXCITATION : spsExcitationSystemLib/Excitation System  tr=20e-3  reg=[ 200, 0.001 ]  exc=[ 1, 0 ]  tgr=[ 0, 0 ]  damp=[ 0.001, 0.1 ]  sat=[ 0, 0 ]  lim="[ 0,  7, 0 ]"  v0=[1 1.4817]
      settings: LibrarySourceBlock=sps_lib/Electrical Machines/Synchronous Machine Control/Excitation System
  Generic Power System Stabilizer : spsGenericPowerSystemStabilizerLib/Generic Power System Stabilizer  Tsensor=15e-3  K=2  Twashout=0.7  Tleadlag1="[60e-3  0.5]"  Tleadlag2=[0 0]  VSlimits=[-0.15 0.15]  Vinit=0  Plot_On=off  MagdB_On=on  FreqRange=logspace(-2,2,500)
      settings: LibrarySourceBlock=|
      | sps_lib/Electrical Machines/Synchronous Machine Control/Generic
      | Power System Stabilizer
  HTG : spsHydraulicTurbineandGovernorLib/Hydraulic Turbine and Governor  sm="[ 10/3  0.07 ]"  gate="[  0.01  0.97518  -0.1  0.1 ]"  reg="[  0.05  1.163  0.105  0  0.01  ]"  hyd="[  0  2.67  ]"  dref=0  po=0.827
      settings: LibrarySourceBlock=|
      | sps_lib/Electrical Machines/Synchronous Machine Control/Hydraulic Turbine
      | and Governor
  Multi-Band Power System Stabilizer : spsMultiBandPowerSystemStabilizerLib/Multi-Band Power System Stabilizer  OperationMode=Simplified settings  Kg=1.0  GL=[0.025 5]  GI=[0.8 25]  GH=[12.0 145]  GLd=[66 66 9.4]  TcLF=[1.667 2 0 0 0 0 2 2.4 0 0 0 0 1 1]  GId=[66 66 47.6]  TcIF=[1 1 0.25 0.3 0 0 1 1 0.3 0.36 0 0 0 0]  GHd=[66 66 233]  TcHF="[0.01 0.012 0 0 0 0  0.012 0.0144 0 0 0 0 1 1]"  LIM=[.075 .15 .15 .15]  Plot_On=off  MagdB_On=off  FreqRange=logspace(-2,2,500)
      settings: LibrarySourceBlock=|
      | sps_lib/Electrical Machines/Synchronous Machine Control/Multi-Band
      | Power System Stabilizer
  Multiport Switch : MultiPortSwitch  InputSameDT=off
  PSS : Constant
  Real-Imag to Complex : RealImagToComplex
  Sum : Sum  SaturateOnIntegerOverflow=on
  Sum2 : Sum  Inputs=-+  InputSameDT=on  SaturateOnIntegerOverflow=on  OutDataTypeStr=Inherit: Same as first input
  Terminator : Terminator
  Vref1 : Constant
  no PSS : Constant  Value=0
  wref : Constant
  Pm : Outport  InitialOutput=0  VectorParamsAs1DForOutWhenUnconnected=off
  Vf : Outport  Port=2  InitialOutput=0  VectorParamsAs1DForOutWhenUnconnected=off
  tag scope: Vt1=global, d_theta1=global, w1=global
  wires:
  Real-Imag to Complex/1 -> Complex to Magnitude-Angle/1
  HTG/2 -> Terminator/1
  Vref1/1 -> EXCITATION/1
  m/1 -> Bus Selector/1
  Bus Selector/5 -> HTG/5, Multi-Band Power System Stabilizer/1  "<Rotor speed deviation  dw (pu)>"
  Bus Selector/4 -> HTG/3, [w1]  "<Rotor speed  wm  (pu)>"
  Pref/1 -> HTG/2
  wref/1 -> HTG/1
  HTG/1 -> Pm/1, Sum2/2
  Bus Selector/2 -> Real-Imag to Complex/2, EXCITATION/3  "<Stator voltage  vq (pu)>"
  EXCITATION/1 -> Vf/1
  Bus Selector/1 -> Real-Imag to Complex/1, EXCITATION/2  "<Stator voltage  vd (pu)>"
  Complex to Magnitude-Angle/1 -> [Vt1]
  Bus Selector/3 -> [d_theta1]  "<Rotor angle deviation  d_theta (rad)>"
  Sum2/1 -> Generic Power System Stabilizer/1  "Pa = Pm-Pe"
  Generic Power System Stabilizer/1 -> Multiport Switch/3
  Multi-Band Power System Stabilizer/1 -> Multiport Switch/4
  no PSS/1 -> Multiport Switch/2
  Multiport Switch/1 -> EXCITATION/4
  [PSS] -> Sum/1
  PSS/1 -> Sum/2
  Sum/1 -> Multiport Switch/1
  Bus Selector/6 -> HTG/4, Sum2/1  "<Output active power   Peo (pu)>"

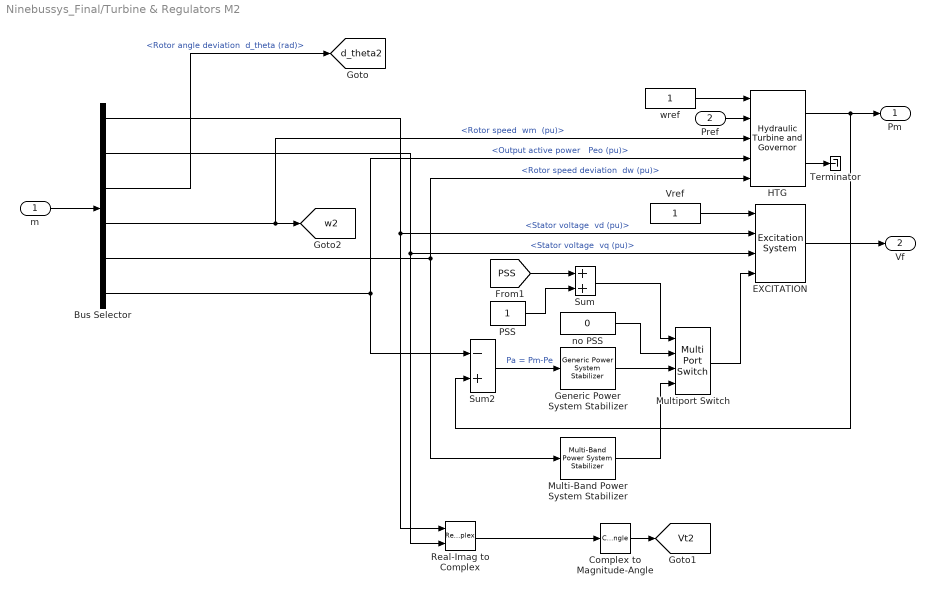
== system Ninebussys_Final/Turbine & Regulators M2 ==
  m : Inport
  Pref : Inport  Port=2
  Bus Selector : BusSelector  OutputSignals="dq0 components.Stator voltage  vd (pu),dq0 components.Stator voltage  vq (pu),Mechanical.Rotor angle deviation  d_theta (rad),Mechanical.Rotor speed  wm  (pu),Mechanical.Rotor speed deviation  dw (pu),Output active power   Peo (pu)"
  Complex to Magnitude-Angle : ComplexToMagnitudeAngle  Output=Magnitude
  EXCITATION : spsExcitationSystemLib/Excitation System  tr=20e-3  reg=[ 200, 0.001 ]  exc=[ 1, 0 ]  tgr=[ 0, 0 ]  damp=[ 0.001, 0.1 ]  sat=[ 0, 0 ]  lim="[ 0,  7, 0 ]"  v0=[1 1.3662]
      settings: LibrarySourceBlock=sps_lib/Electrical Machines/Synchronous Machine Control/Excitation System
  Generic Power System Stabilizer : spsGenericPowerSystemStabilizerLib/Generic Power System Stabilizer  Tsensor=15e-3  K=2  Twashout=0.7  Tleadlag1="[60e-3  0.5]"  Tleadlag2=[0 0]  VSlimits=[-0.15 0.15]  Vinit=0  Plot_On=off  MagdB_On=on  FreqRange=logspace(-2,2,500)
      settings: LibrarySourceBlock=|
      | sps_lib/Electrical Machines/Synchronous Machine Control/Generic
      | Power System Stabilizer
  HTG : spsHydraulicTurbineandGovernorLib/Hydraulic Turbine and Governor  sm="[ 10/3  0.07 ]"  gate="[  0.01  0.97518  -0.1  0.1 ]"  reg="[  0.05  1.163  0.105  0  0.01  ]"  hyd="[  0  2.67  ]"  dref=0  po=0.63993
      settings: LibrarySourceBlock=|
      | sps_lib/Electrical Machines/Synchronous Machine Control/Hydraulic Turbine
      | and Governor
  Multi-Band Power System Stabilizer : spsMultiBandPowerSystemStabilizerLib/Multi-Band Power System Stabilizer  OperationMode=Simplified settings  Kg=1.0  GL=[0.025 5]  GI=[0.8 25]  GH=[12.0 145]  GLd=[66 66 9.4]  TcLF=[1.667 2 0 0 0 0 2 2.4 0 0 0 0 1 1]  GId=[66 66 47.6]  TcIF=[1 1 0.25 0.3 0 0 1 1 0.3 0.36 0 0 0 0]  GHd=[66 66 233]  TcHF="[0.01 0.012 0 0 0 0  0.012 0.0144 0 0 0 0 1 1]"  LIM=[.075 .15 .15 .15]  Plot_On=off  MagdB_On=off  FreqRange=logspace(-2,2,500)
      settings: LibrarySourceBlock=|
      | sps_lib/Electrical Machines/Synchronous Machine Control/Multi-Band
      | Power System Stabilizer
  Multiport Switch : MultiPortSwitch  InputSameDT=off
  PSS : Constant
  Real-Imag to Complex : RealImagToComplex
  Sum : Sum  SaturateOnIntegerOverflow=on
  Sum2 : Sum  Inputs=-+  InputSameDT=on  SaturateOnIntegerOverflow=on  OutDataTypeStr=Inherit: Same as first input
  Terminator : Terminator
  Vref : Constant
  no PSS : Constant  Value=0
  wref : Constant
  Pm : Outport  InitialOutput=0  VectorParamsAs1DForOutWhenUnconnected=off
  Vf : Outport  Port=2  InitialOutput=0  VectorParamsAs1DForOutWhenUnconnected=off
  tag scope: Vt2=global, d_theta2=global, w2=global
  wires:
  PSS/1 -> Sum/2
  [PSS] -> Sum/1
  Real-Imag to Complex/1 -> Complex to Magnitude-Angle/1
  HTG/2 -> Terminator/1
  Vref/1 -> EXCITATION/1
  m/1 -> Bus Selector/1
  Bus Selector/5 -> HTG/5, Multi-Band Power System Stabilizer/1  "<Rotor speed deviation  dw (pu)>"
  Bus Selector/6 -> Sum2/1, HTG/4  "<Output active power   Peo (pu)>"
  Bus Selector/4 -> [w2], HTG/3  "<Rotor speed  wm  (pu)>"
  Pref/1 -> HTG/2
  wref/1 -> HTG/1
  HTG/1 -> Pm/1, Sum2/2
  Bus Selector/2 -> Real-Imag to Complex/2, EXCITATION/3  "<Stator voltage  vq (pu)>"
  EXCITATION/1 -> Vf/1
  Bus Selector/1 -> Real-Imag to Complex/1, EXCITATION/2  "<Stator voltage  vd (pu)>"
  Complex to Magnitude-Angle/1 -> [Vt2]
  Bus Selector/3 -> [d_theta2]  "<Rotor angle deviation  d_theta (rad)>"
  Sum2/1 -> Generic Power System Stabilizer/1  "Pa = Pm-Pe"
  Generic Power System Stabilizer/1 -> Multiport Switch/3
  Multi-Band Power System Stabilizer/1 -> Multiport Switch/4
  no PSS/1 -> Multiport Switch/2
  Sum/1 -> Multiport Switch/1
  Multiport Switch/1 -> EXCITATION/4

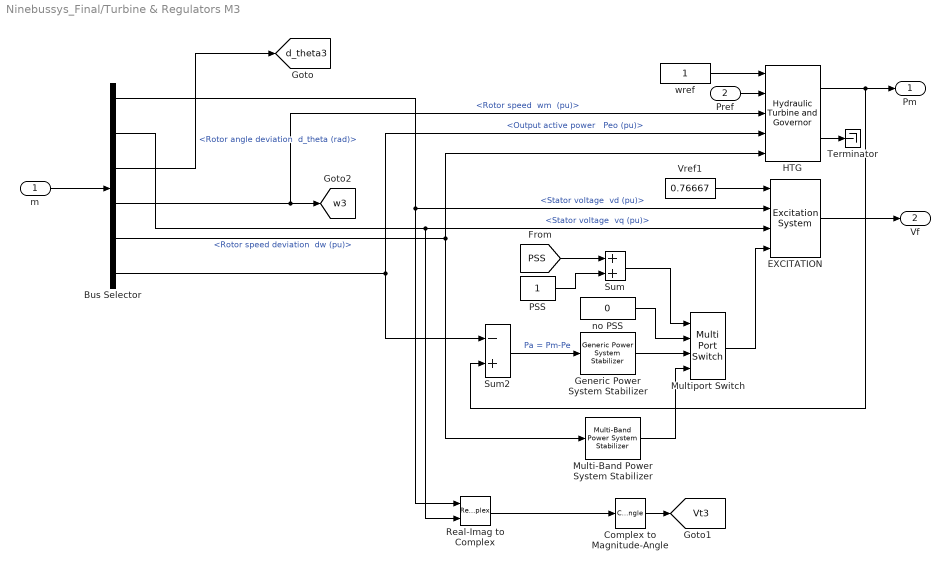
== system Ninebussys_Final/Turbine & Regulators M3 ==
  m : Inport
  Pref : Inport  Port=2
  Bus Selector : BusSelector  OutputSignals="dq0 components.Stator voltage  vd (pu),dq0 components.Stator voltage  vq (pu),Mechanical.Rotor angle deviation  d_theta (rad),Mechanical.Rotor speed  wm  (pu),Mechanical.Rotor speed deviation  dw (pu),Output active power   Peo (pu)"
  Complex to Magnitude-Angle : ComplexToMagnitudeAngle  Output=Magnitude
  EXCITATION : spsExcitationSystemLib/Excitation System  tr=20e-3  reg=[ 200, 0.001 ]  exc=[ 1, 0 ]  tgr=[ 0, 0 ]  damp=[ 0.001, 0.1 ]  sat=[ 0, 0 ]  lim="[ 0,  7, 0 ]"  v0=[0.76667 1.0466]
      settings: LibrarySourceBlock=sps_lib/Electrical Machines/Synchronous Machine Control/Excitation System
  Generic Power System Stabilizer : spsGenericPowerSystemStabilizerLib/Generic Power System Stabilizer  Tsensor=15e-3  K=2  Twashout=0.7  Tleadlag1="[60e-3  0.5]"  Tleadlag2=[0 0]  VSlimits=[-0.15 0.15]  Vinit=0  Plot_On=off  MagdB_On=on  FreqRange=logspace(-2,2,500)
      settings: LibrarySourceBlock=|
      | sps_lib/Electrical Machines/Synchronous Machine Control/Generic
      | Power System Stabilizer
  HTG : spsHydraulicTurbineandGovernorLib/Hydraulic Turbine and Governor  sm="[ 10/3  0.07 ]"  gate="[  0.01  0.97518  -0.1  0.1 ]"  reg="[  0.05  1.163  0.105  0  0.01  ]"  hyd="[  0  2.67  ]"  dref=0  po=0.42589
      settings: LibrarySourceBlock=|
      | sps_lib/Electrical Machines/Synchronous Machine Control/Hydraulic Turbine
      | and Governor
  Multi-Band Power System Stabilizer : spsMultiBandPowerSystemStabilizerLib/Multi-Band Power System Stabilizer  OperationMode=Simplified settings  Kg=1.0  GL=[0.025 5]  GI=[0.8 25]  GH=[12.0 145]  GLd=[66 66 9.4]  TcLF=[1.667 2 0 0 0 0 2 2.4 0 0 0 0 1 1]  GId=[66 66 47.6]  TcIF=[1 1 0.25 0.3 0 0 1 1 0.3 0.36 0 0 0 0]  GHd=[66 66 233]  TcHF="[0.01 0.012 0 0 0 0  0.012 0.0144 0 0 0 0 1 1]"  LIM=[.075 .15 .15 .15]  Plot_On=off  MagdB_On=off  FreqRange=logspace(-2,2,500)
      settings: LibrarySourceBlock=|
      | sps_lib/Electrical Machines/Synchronous Machine Control/Multi-Band
      | Power System Stabilizer
  Multiport Switch : MultiPortSwitch  InputSameDT=off
  PSS : Constant
  Real-Imag to Complex : RealImagToComplex
  Sum : Sum  SaturateOnIntegerOverflow=on
  Sum2 : Sum  Inputs=-+  InputSameDT=on  SaturateOnIntegerOverflow=on  OutDataTypeStr=Inherit: Same as first input
  Terminator : Terminator
  Vref1 : Constant  Value=0.76667
  no PSS : Constant  Value=0
  wref : Constant
  Pm : Outport  InitialOutput=0  VectorParamsAs1DForOutWhenUnconnected=off
  Vf : Outport  Port=2  InitialOutput=0  VectorParamsAs1DForOutWhenUnconnected=off
  tag scope: Vt3=global, d_theta3=global, w3=global
  wires:
  Real-Imag to Complex/1 -> Complex to Magnitude-Angle/1
  HTG/2 -> Terminator/1
  Vref1/1 -> EXCITATION/1
  m/1 -> Bus Selector/1
  Bus Selector/5 -> HTG/5, Multi-Band Power System Stabilizer/1  "<Rotor speed deviation  dw (pu)>"
  Bus Selector/4 -> HTG/3, [w3]  "<Rotor speed  wm  (pu)>"
  Pref/1 -> HTG/2
  wref/1 -> HTG/1
  HTG/1 -> Pm/1, Sum2/2
  Bus Selector/2 -> Real-Imag to Complex/2, EXCITATION/3  "<Stator voltage  vq (pu)>"
  EXCITATION/1 -> Vf/1
  Bus Selector/1 -> Real-Imag to Complex/1, EXCITATION/2  "<Stator voltage  vd (pu)>"
  Complex to Magnitude-Angle/1 -> [Vt3]
  Bus Selector/3 -> [d_theta3]  "<Rotor angle deviation  d_theta (rad)>"
  Sum2/1 -> Generic Power System Stabilizer/1  "Pa = Pm-Pe"
  Generic Power System Stabilizer/1 -> Multiport Switch/3
  Multi-Band Power System Stabilizer/1 -> Multiport Switch/4
  no PSS/1 -> Multiport Switch/2
  Multiport Switch/1 -> EXCITATION/4
  [PSS] -> Sum/1
  PSS/1 -> Sum/2
  Sum/1 -> Multiport Switch/1
  Bus Selector/6 -> HTG/4, Sum2/1  "<Output active power   Peo (pu)>"

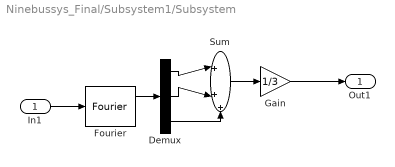
== system Ninebussys_Final/Subsystem1/Subsystem ==
  In1 : Inport
  Demux : Demux  Outputs=3
  Fourier : spsFourierLib/Fourier  Freq=50  n=1  InInit=[0, 0]  Ts=50e-6
  Gain : Gain  Gain=1/3
  Sum : Sum  Inputs=|+++
  Out1 : Outport  VectorParamsAs1DForOutWhenUnconnected=off
  wires:
  In1/1 -> Fourier/1
  Demux/1 -> Sum/1
  Demux/3 -> Sum/3
  Sum/1 -> Gain/1
  Gain/1 -> Out1/1
  Demux/2 -> Sum/2
  Fourier/1 -> Demux/1

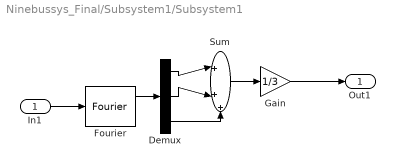
== system Ninebussys_Final/Subsystem1/Subsystem1 ==
  In1 : Inport
  Demux : Demux  Outputs=3
  Fourier : spsFourierLib/Fourier  Freq=50  n=1  InInit=[0, 0]  Ts=50e-6
  Gain : Gain  Gain=1/3
  Sum : Sum  Inputs=|+++
  Out1 : Outport  VectorParamsAs1DForOutWhenUnconnected=off
  wires:
  Fourier/1 -> Demux/1
  Demux/2 -> Sum/2
  Gain/1 -> Out1/1
  Sum/1 -> Gain/1
  Demux/3 -> Sum/3
  Demux/1 -> Sum/1
  In1/1 -> Fourier/1

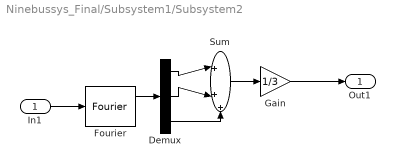
== system Ninebussys_Final/Subsystem1/Subsystem2 ==
  In1 : Inport
  Demux : Demux  Outputs=3
  Fourier : spsFourierLib/Fourier  Freq=50  n=1  InInit=[0, 0]  Ts=50e-6
  Gain : Gain  Gain=1/3
  Sum : Sum  Inputs=|+++
  Out1 : Outport  VectorParamsAs1DForOutWhenUnconnected=off
  wires:
  Fourier/1 -> Demux/1
  Demux/2 -> Sum/2
  Gain/1 -> Out1/1
  Sum/1 -> Gain/1
  Demux/3 -> Sum/3
  Demux/1 -> Sum/1
  In1/1 -> Fourier/1

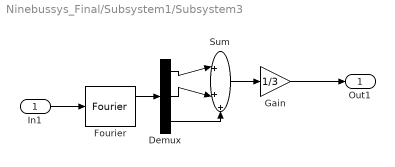
== system Ninebussys_Final/Subsystem1/Subsystem3 ==
  In1 : Inport
  Demux : Demux  Outputs=3
  Fourier : spsFourierLib/Fourier  Freq=50  n=1  InInit=[0, 0]  Ts=50e-6
  Gain : Gain  Gain=1/3
  Sum : Sum  Inputs=|+++
  Out1 : Outport  VectorParamsAs1DForOutWhenUnconnected=off
  wires:
  In1/1 -> Fourier/1
  Demux/1 -> Sum/1
  Demux/3 -> Sum/3
  Sum/1 -> Gain/1
  Gain/1 -> Out1/1
  Demux/2 -> Sum/2
  Fourier/1 -> Demux/1

== system Ninebussys_Final/Subsystem1/Subsystem4 ==
  In1 : Inport
  Demux : Demux  Outputs=3
  Fourier : spsFourierLib/Fourier  Freq=50  n=1  InInit=[0, 0]  Ts=50e-6
  Gain : Gain  Gain=1/3
  Sum : Sum  Inputs=|+++
  Out1 : Outport  VectorParamsAs1DForOutWhenUnconnected=off
  wires:
  Fourier/1 -> Demux/1
  Demux/2 -> Sum/2
  Gain/1 -> Out1/1
  Sum/1 -> Gain/1
  Demux/3 -> Sum/3
  Demux/1 -> Sum/1
  In1/1 -> Fourier/1

== system Ninebussys_Final/Subsystem1/Subsystem5 ==
  In1 : Inport
  Demux : Demux  Outputs=3
  Fourier : spsFourierLib/Fourier  Freq=50  n=1  InInit=[0, 0]  Ts=50e-6
  Gain : Gain  Gain=1/3
  Sum : Sum  Inputs=|+++
  Out1 : Outport  VectorParamsAs1DForOutWhenUnconnected=off
  wires:
  In1/1 -> Fourier/1
  Demux/1 -> Sum/1
  Demux/3 -> Sum/3
  Sum/1 -> Gain/1
  Gain/1 -> Out1/1
  Demux/2 -> Sum/2
  Fourier/1 -> Demux/1

== system Ninebussys_Final/Subsystem1/Subsystem6 ==
  In1 : Inport
  Demux : Demux  Outputs=3
  Fourier : spsFourierLib/Fourier  Freq=50  n=1  InInit=[0, 0]  Ts=50e-6
  Gain : Gain  Gain=1/3
  Sum : Sum  Inputs=|+++
  Out1 : Outport  VectorParamsAs1DForOutWhenUnconnected=off
  wires:
  In1/1 -> Fourier/1
  Demux/1 -> Sum/1
  Demux/3 -> Sum/3
  Sum/1 -> Gain/1
  Gain/1 -> Out1/1
  Demux/2 -> Sum/2
  Fourier/1 -> Demux/1

== system Ninebussys_Final/Subsystem1/Subsystem7 ==
  In1 : Inport
  Demux : Demux  Outputs=3
  Fourier : spsFourierLib/Fourier  Freq=50  n=1  InInit=[0, 0]  Ts=50e-6
  Gain : Gain  Gain=1/3
  Sum : Sum  Inputs=|+++
  Out1 : Outport  VectorParamsAs1DForOutWhenUnconnected=off
  wires:
  Fourier/1 -> Demux/1
  Demux/2 -> Sum/2
  Gain/1 -> Out1/1
  Sum/1 -> Gain/1
  Demux/3 -> Sum/3
  Demux/1 -> Sum/1
  In1/1 -> Fourier/1

== system Ninebussys_Final/Subsystem1/Subsystem8 ==
  In1 : Inport
  Demux : Demux  Outputs=3
  Fourier : spsFourierLib/Fourier  Freq=50  n=1  InInit=[0, 0]  Ts=50e-6
  Gain : Gain  Gain=1/3
  Sum : Sum  Inputs=|+++
  Out1 : Outport  VectorParamsAs1DForOutWhenUnconnected=off
  wires:
  In1/1 -> Fourier/1
  Demux/1 -> Sum/1
  Demux/3 -> Sum/3
  Sum/1 -> Gain/1
  Gain/1 -> Out1/1
  Demux/2 -> Sum/2
  Fourier/1 -> Demux/1

== system Ninebussys_Final/Subsystem2/Subsystem ==
  In1 : Inport
  Demux : Demux  Outputs=3
  Fourier : spsFourierLib/Fourier  Freq=50  n=1  InInit=[0, 0]  Ts=50e-6
  Gain : Gain  Gain=1/3
  Sum : Sum  Inputs=|+++
  Out1 : Outport  VectorParamsAs1DForOutWhenUnconnected=off
  wires:
  Fourier/1 -> Demux/1
  Demux/2 -> Sum/2
  Gain/1 -> Out1/1
  Sum/1 -> Gain/1
  Demux/3 -> Sum/3
  Demux/1 -> Sum/1
  In1/1 -> Fourier/1

== system Ninebussys_Final/Subsystem2/Subsystem1 ==
  In1 : Inport
  Demux : Demux  Outputs=3
  Fourier : spsFourierLib/Fourier  Freq=50  n=1  InInit=[0, 0]  Ts=50e-6
  Gain : Gain  Gain=1/3
  Sum : Sum  Inputs=|+++
  Out1 : Outport  VectorParamsAs1DForOutWhenUnconnected=off
  wires:
  In1/1 -> Fourier/1
  Demux/1 -> Sum/1
  Demux/3 -> Sum/3
  Sum/1 -> Gain/1
  Gain/1 -> Out1/1
  Demux/2 -> Sum/2
  Fourier/1 -> Demux/1

== system Ninebussys_Final/Subsystem2/Subsystem2 ==
  In1 : Inport
  Demux : Demux  Outputs=3
  Fourier : spsFourierLib/Fourier  Freq=50  n=1  InInit=[0, 0]  Ts=50e-6
  Gain : Gain  Gain=1/3
  Sum : Sum  Inputs=|+++
  Out1 : Outport  VectorParamsAs1DForOutWhenUnconnected=off
  wires:
  In1/1 -> Fourier/1
  Demux/1 -> Sum/1
  Demux/3 -> Sum/3
  Sum/1 -> Gain/1
  Gain/1 -> Out1/1
  Demux/2 -> Sum/2
  Fourier/1 -> Demux/1

== system Ninebussys_Final/Subsystem2/Subsystem3 ==
  In1 : Inport
  Demux : Demux  Outputs=3
  Fourier : spsFourierLib/Fourier  Freq=50  n=1  InInit=[0, 0]  Ts=50e-6
  Gain : Gain  Gain=1/3
  Sum : Sum  Inputs=|+++
  Out1 : Outport  VectorParamsAs1DForOutWhenUnconnected=off
  wires:
  Fourier/1 -> Demux/1
  Demux/2 -> Sum/2
  Gain/1 -> Out1/1
  Sum/1 -> Gain/1
  Demux/3 -> Sum/3
  Demux/1 -> Sum/1
  In1/1 -> Fourier/1

== system Ninebussys_Final/Subsystem2/Subsystem4 ==
  In1 : Inport
  Demux : Demux  Outputs=3
  Fourier : spsFourierLib/Fourier  Freq=50  n=1  InInit=[0, 0]  Ts=50e-6
  Gain : Gain  Gain=1/3
  Sum : Sum  Inputs=|+++
  Out1 : Outport  VectorParamsAs1DForOutWhenUnconnected=off
  wires:
  In1/1 -> Fourier/1
  Demux/1 -> Sum/1
  Demux/3 -> Sum/3
  Sum/1 -> Gain/1
  Gain/1 -> Out1/1
  Demux/2 -> Sum/2
  Fourier/1 -> Demux/1

== system Ninebussys_Final/Subsystem2/Subsystem5 ==
  In1 : Inport
  Demux : Demux  Outputs=3
  Fourier : spsFourierLib/Fourier  Freq=50  n=1  InInit=[0, 0]  Ts=50e-6
  Gain : Gain  Gain=1/3
  Sum : Sum  Inputs=|+++
  Out1 : Outport  VectorParamsAs1DForOutWhenUnconnected=off
  wires:
  Fourier/1 -> Demux/1
  Demux/2 -> Sum/2
  Gain/1 -> Out1/1
  Sum/1 -> Gain/1
  Demux/3 -> Sum/3
  Demux/1 -> Sum/1
  In1/1 -> Fourier/1

== system Ninebussys_Final/Subsystem2/Subsystem6 ==
  In1 : Inport
  Demux : Demux  Outputs=3
  Fourier : spsFourierLib/Fourier  Freq=50  n=1  InInit=[0, 0]  Ts=50e-6
  Gain : Gain  Gain=1/3
  Sum : Sum  Inputs=|+++
  Out1 : Outport  VectorParamsAs1DForOutWhenUnconnected=off
  wires:
  Fourier/1 -> Demux/1
  Demux/2 -> Sum/2
  Gain/1 -> Out1/1
  Sum/1 -> Gain/1
  Demux/3 -> Sum/3
  Demux/1 -> Sum/1
  In1/1 -> Fourier/1

== system Ninebussys_Final/Subsystem2/Subsystem7 ==
  In1 : Inport
  Demux : Demux  Outputs=3
  Fourier : spsFourierLib/Fourier  Freq=50  n=1  InInit=[0, 0]  Ts=50e-6
  Gain : Gain  Gain=1/3
  Sum : Sum  Inputs=|+++
  Out1 : Outport  VectorParamsAs1DForOutWhenUnconnected=off
  wires:
  In1/1 -> Fourier/1
  Demux/1 -> Sum/1
  Demux/3 -> Sum/3
  Sum/1 -> Gain/1
  Gain/1 -> Out1/1
  Demux/2 -> Sum/2
  Fourier/1 -> Demux/1

== system Ninebussys_Final/Subsystem2/Subsystem8 ==
  In1 : Inport
  Demux : Demux  Outputs=3
  Fourier : spsFourierLib/Fourier  Freq=50  n=1  InInit=[0, 0]  Ts=50e-6
  Gain : Gain  Gain=1/3
  Sum : Sum  Inputs=|+++
  Out1 : Outport  VectorParamsAs1DForOutWhenUnconnected=off
  wires:
  Fourier/1 -> Demux/1
  Demux/2 -> Sum/2
  Gain/1 -> Out1/1
  Sum/1 -> Gain/1
  Demux/3 -> Sum/3
  Demux/1 -> Sum/1
  In1/1 -> Fourier/1
